simulink model "free"  (Simulink 8.1)
settings: Solver=ode45  StartTime=0.0  StopTime=1500  RelTol=1e-3
settings Model: Creator=kr2112  LastModifiedBy=spikelucky
settings DebuggingCC: FcnCallInpInsideContextMsg=EnableAllAsWarning
settings GRTTargetCC: CombineOutputUpdateFcns=on  GRTInterface=off

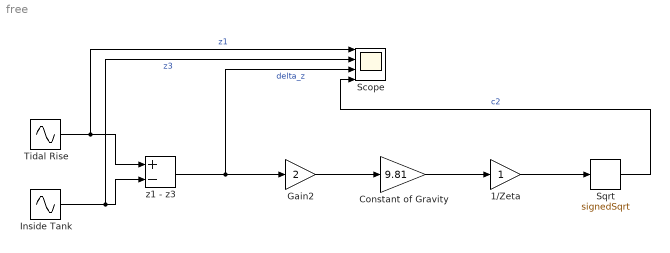
== system free ==
  1/Zeta : Gain
  Constant of Gravity : Gain  Gain=9.81
  Gain2 : Gain  Gain=2
  Inside Tank : Sin  Frequency=0.0083  Phase=-pi/16  SampleTime=0
  Scope : Scope  NumInputPorts=4
      settings: YMin=-5~-5~-5~-5  YMax=5~5~5~5
  Sqrt : Sqrt  Operator=signedSqrt  SaturateOnIntegerOverflow=on
  Tidal Rise : Sin  Frequency=0.0083  SampleTime=0
  z1 - z3 : Sum  Inputs=+-
  wires:
  Constant of Gravity/1 -> 1/Zeta/1
  Sqrt/1 -> Scope/4  "c2"
  z1 - z3/1 -> Scope/3, Gain2/1  "delta_z"
  Tidal Rise/1 -> z1 - z3/1, Scope/1  "z1"
  Inside Tank/1 -> z1 - z3/2, Scope/2  "z3"
  Gain2/1 -> Constant of Gravity/1
  1/Zeta/1 -> Sqrt/1
